simulink model "L11Sim"  (R2020b)
settings: Solver=VariableStepAuto  StartTime=0.0  StopTime=10.0  RelTol=1e-3
values from neighbouring files (symbols this model uses):
  a = 0.99    [L11.m]
settings Model: Creator=Nic  LastModifiedBy=Nic

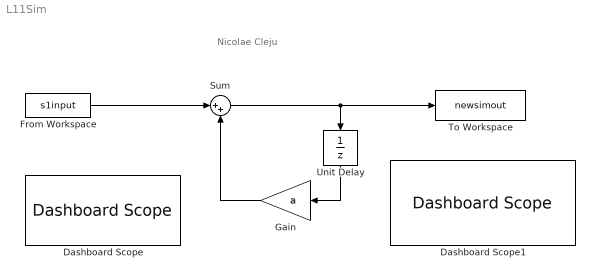
== system L11Sim ==
  note: Nicolae Cleju
  Dashboard Scope : DashboardScope
  Dashboard Scope1 : DashboardScope
  From Workspace : FromWorkspace  VariableName=s1input  SampleTime=0.001
  Gain : Gain  Gain=a
  Sum : Sum  Inputs=|++
  To Workspace : ToWorkspace  VariableName=newsimout  SampleTime=-1
  Unit Delay : UnitDelay  SampleTime=-1  HasFrameUpgradeWarning=on
  wires:
  Sum/1 -> To Workspace/1, Unit Delay/1
  Unit Delay/1 -> Gain/1
  Gain/1 -> Sum/2
  From Workspace/1 -> Sum/1
